simulink model "lab6_simulink"  (R2021b)
settings: Solver=VariableStepAuto  StartTime=0.0  StopTime=24.0  RelTol=1e-3
values from neighbouring files (symbols this model uses):
  Cd = ss_d.C    [lab12.m]
  F = ss_d.A    [lab12.m]
  H = ss_d.B    [lab12.m]
undefined symbols (not defined in the file or in its folder): L_T, p_d_con
settings Model: Creator=11760739  LastModifiedBy=11892153

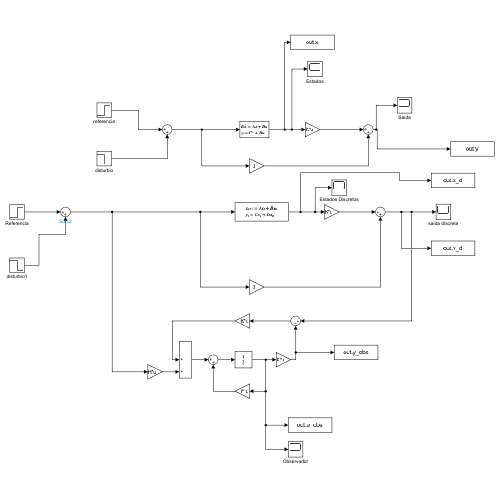
[thumbnail: Simulink's stored preview of the top-level diagram]
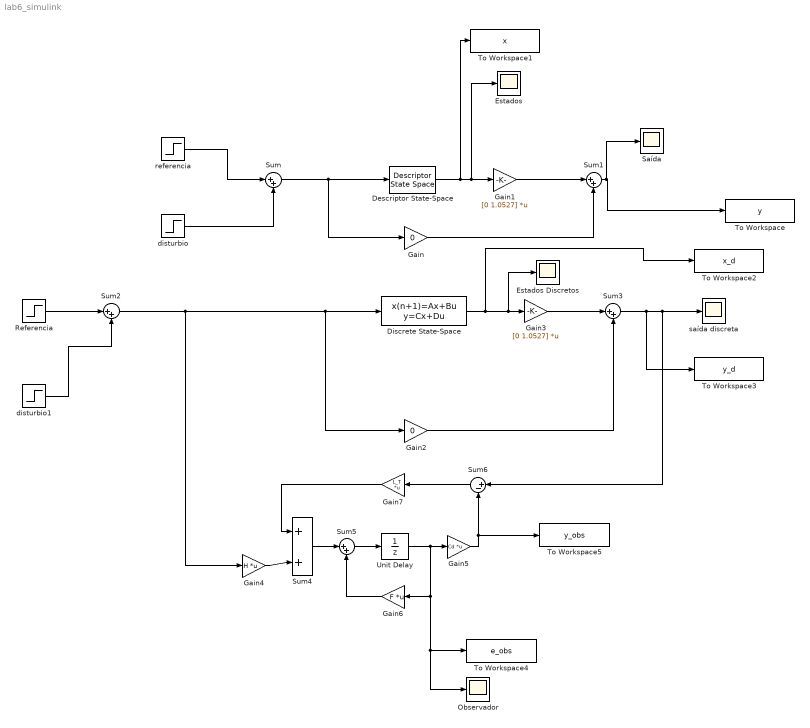
== system lab6_simulink ==
  Descriptor State-Space : DescriptorStateSpace  E=[1 0; 0 1]  A=[-2.0787 -1.0527; 1 0]  B=[1; 0]  C=[1 0; 0 1]  D=[0; 0]
  Discrete State-Space : DiscreteStateSpace  A=[0.3007 -0.3089; 0.2934 0.9107]  B=[0.2934; 0.0848]  C=[1 0; 0 1]  D=[0; 0]  InitialCondition=p_d_con  SampleTime=0.4855
  Estados : Scope
  Estados Discretos : Scope
  Gain : Gain  Gain=0
  Gain1 : Gain  Gain=[0 1.0527]  Multiplication=Matrix(K*u)
  Gain2 : Gain  Gain=0
  Gain3 : Gain  Gain=[0 1.0527]  Multiplication=Matrix(K*u)
  Gain4 : Gain  Gain=H  Multiplication=Matrix(K*u)
  Gain5 : Gain  Gain=Cd  Multiplication=Matrix(K*u)
  Gain6 : Gain  Gain=F  Multiplication=Matrix(K*u)
  Gain7 : Gain  Gain=L_T  Multiplication=Matrix(K*u)
  Observador : Scope
  Referencia : Step  Time=0  After=1.18  SampleTime=0
  Saída : Scope
  Sum{,1..5} (6 alike) : Sum  Inputs=|++
  Sum6 : Sum  Inputs=|+-
  To Workspace : ToWorkspace  VariableName=y  SaveFormat=Timeseries  SampleTime=-1
  To Workspace1 : ToWorkspace  VariableName=x  SaveFormat=Timeseries  SampleTime=-1
  To Workspace2 : ToWorkspace  VariableName=x_d  SaveFormat=Timeseries  SampleTime=-1
  To Workspace3 : ToWorkspace  VariableName=y_d  SaveFormat=Timeseries  SampleTime=-1
  To Workspace4 : ToWorkspace  VariableName=e_obs  SaveFormat=Timeseries  SampleTime=-1
  To Workspace5 : ToWorkspace  VariableName=y_obs  SaveFormat=Timeseries  SampleTime=-1
  Unit Delay : UnitDelay  InitialCondition=[0 0]  SampleTime=-1  HasFrameUpgradeWarning=on
  disturbio : Step  Time=15  After=-0.13  SampleTime=0
  disturbio1 : Step  Time=15  After=-0.13  SampleTime=0
  referencia : Step  Time=0  After=1.18  SampleTime=0
  saída discreta : Scope
  wires:
  Sum/1 -> Gain/1, Descriptor State-Space/1
  disturbio/1 -> Sum/2
  referencia/1 -> Sum/1
  Descriptor State-Space/1 -> To Workspace1/1, Estados/1, Gain1/1
  Gain1/1 -> Sum1/1
  Gain/1 -> Sum1/2
  Referencia/1 -> Sum2/1
  disturbio1/1 -> Sum2/2
  Sum2/1 -> Gain4/1, Discrete State-Space/1, Gain2/1
  Gain3/1 -> Sum3/1
  Gain2/1 -> Sum3/2
  Sum3/1 -> Sum6/1, saída discreta/1, To Workspace3/1
  Unit Delay/1 -> To Workspace4/1, Observador/1, Gain6/1, Gain5/1
  Sum4/1 -> Sum5/1
  Sum5/1 -> Unit Delay/1
  Gain6/1 -> Sum5/2
  Gain5/1 -> To Workspace5/1, Sum6/2
  Sum6/1 -> Gain7/1
  Gain7/1 -> Sum4/1
  Gain4/1 -> Sum4/2
  Sum1/1 -> Saída/1, To Workspace/1
  Discrete State-Space/1 -> To Workspace2/1, Estados Discretos/1, Gain3/1
